simulink model "pp_sim"  (R2025a)
settings: Solver=VariableStepAuto  StartTime=0.0  StopTime=40  RelTol=1e-3
model workspace (MAT data in the model file):
  p_m = 0
  v_f = 0.8705
libraries: spsGroundLib x3, spsThreePhaseVIMeasurementLib x3, spsThreePhaseBreakerLib x3, spsSynchronousMachinepuFundamentalLib x2, spsThreePhaseProgrammableVoltageSourceLib x2, spsThreePhaseParallelRLCBranchLib x1, spsThreePhaseSourceLib x1, sps_lib x1
settings Model: Creator=reyes  LastModifiedBy=garyr

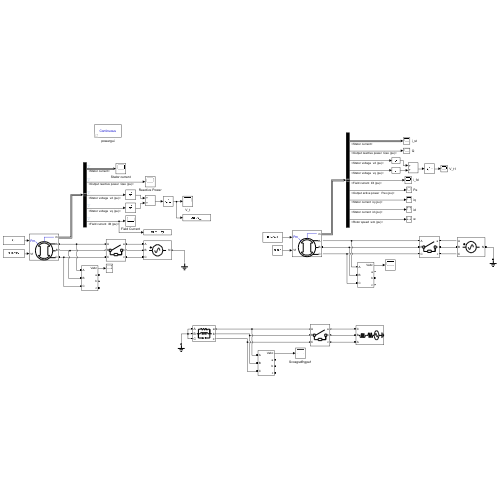
[thumbnail: Simulink's stored preview of the top-level diagram]
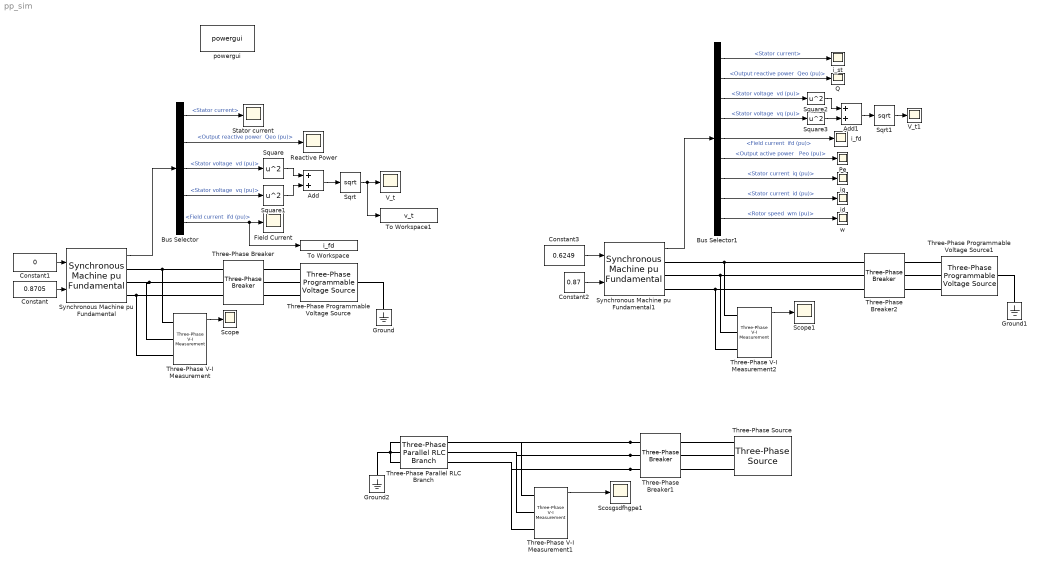
== system pp_sim ==
  Add : Sum
  Add1 : Sum
  Bus Selector : BusSelector  OutputSignals="Stator current,Output reactive power  Qeo (pu),dq0 components.Stator voltage  vd (pu),dq0 components.Stator voltage  vq (pu),dq0 components.Field current  ifd (pu)"
  Bus Selector1 : BusSelector  OutputSignals="Stator current,Output reactive power  Qeo (pu),dq0 components.Stator voltage  vd (pu),dq0 components.Stator voltage  vq (pu),dq0 components.Field current  ifd (pu),Output active power   Peo (pu),dq0 components.Stator current  iq (pu),dq0 components.Stator current  id (pu),Mechanical.Rotor speed  wm (pu)"
  Constant : Constant  Value=0.8705
  Constant1 : Constant  Tag=p_m  Value=0
  Constant2 : Constant  Value=0.87
  Constant3 : Constant  Tag=p_m  Value=0.6249
  Field Current : Scope
      settings: ActiveDisplayYMinimum=0.95426093350087715  ActiveDisplayYMaximum=0.95670423972594421  DataLoggingVariableName=ScopeData4
  Ground : spsGroundLib/Ground  LConnTagsString=a
  Ground1 : spsGroundLib/Ground  LConnTagsString=a
  Ground2 : spsGroundLib/Ground  LConnTagsString=a
  Pe : Scope
      settings: ActiveDisplayYMinimum=-266.63073278249573  ActiveDisplayYMaximum=2375.0722359085885  DataLoggingVariableName=ScopeData11
  Q : Scope
      settings: ActiveDisplayYMinimum=-0.29769400843785104  ActiveDisplayYMaximum=-0.29699694200105431  DataLoggingVariableName=ScopeData7
  Reactive Power : Scope
      settings: ActiveDisplayYMinimum=-0.1233902909232272  ActiveDisplayYMaximum=-0.12338999766576593  DataLoggingVariableName=ScopeData3
  Scope : Scope
      settings: ActiveDisplayYMinimum=-1.2502044389104019  ActiveDisplayYMaximum=1.2500642972287648  DataLoggingVariableName=ScopeData5
  Scope1 : Scope
      settings: ActiveDisplayYMinimum=-1.0713781429903637  ActiveDisplayYMaximum=0.99048701496862079  DataLoggingVariableName=ScopeData8
  Scosgsdfhgpe1 : Scope
      settings: ActiveDisplayYMinimum=-1.0092853712369843  ActiveDisplayYMaximum=1.1869510329971333  DataLoggingVariableName=ScopeData2
  Sqrt : Sqrt
  Sqrt1 : Sqrt
  Square{,1..3} (4 alike) : Math  Operator=square
  Stator current : Scope
      settings: ActiveDisplayYMinimum=0.12291954925426332  ActiveDisplayYMaximum=0.12350538497944295
  Synchronous Machine pu Fundamental : spsSynchronousMachinepuFundamentalLib/Synchronous Machine pu Fundamental  PresetModel=No  MechanicalLoad=Mechanical power Pm  ShowDetailedParameters=on  RotorType=Salient-pole  Units=per unit fundamental parameters  MeasurementBus=off  NominalParameters="[ 6250E3  4160   60]"  Stator="[ 0.00636  0.1235  0.926  0.5078 ]"  Field="[ 0.00084  0.2691]"  Dampers2=[0.0652, 0.5134, 0.0287, 0.2553, 7.765e-3, 0.9167 ]  Dampers1="[ 0.03578  0.1119  0.05366  0.1678 ]"  Mechanical=[ 7.11 0 10]  PolePairs=20  InitialConditions="[ 0  0  0  0  0  0  0  0  1 ]"  SetSaturation=off  Saturation=[0.6404,0.7127,0.8441,0.9214,0.9956,1.082,1.19,1.316,1.457;0.7,0.7698,0.8872,0.9466,0.9969,1.046,1.1,1.151,1.201]  LoadFlowParameters=[1,0,0,0,0]  TsPowergui=0  TsBlock=-1  IterativeModel=Trapezoidal non iterative  IterativeDiscreteModel=Trapezoidal non iterative  BusType=PV  Pref=0  Qref=0.3054  Qmin=-inf  Qmax=inf  PLF=0  QLF=0
      settings: LibrarySourceBlock=|
      | sps_lib/Electrical Machines/Synchronous Machine
      | pu Fundamental
  Synchronous Machine pu Fundamental1 : spsSynchronousMachinepuFundamentalLib/Synchronous Machine pu Fundamental  PresetModel=No  MechanicalLoad=Mechanical power Pm  ShowDetailedParameters=on  RotorType=Salient-pole  Units=per unit fundamental parameters  MeasurementBus=off  NominalParameters="[ 6250E3  4160   60]"  Stator="[ 0.00636  0.1235  0.926  0.5078 ]"  Field="[ 0.0084  0.2691]"  Dampers2=[0.0652, 0.5134, 0.0287, 0.2553, 7.765e-3, 0.9167 ]  Dampers1="[ 0.03578  0.1119  0.05366  0.1678 ]"  Mechanical=[ 7.11 0 20]  PolePairs=20  InitialConditions="[ 0  0  0  0  0  0  0  0  1 ]"  SetSaturation=on  Saturation=[0.6404,0.7127,0.8441,0.9214,0.9956,1.082,1.19,1.316,1.457;0.7,0.7698,0.8872,0.9466,0.9969,1.046,1.1,1.151,1.201]  LoadFlowParameters=[1,0,0,0,0]  TsPowergui=0  TsBlock=-1  IterativeModel=Trapezoidal non iterative  IterativeDiscreteModel=Trapezoidal non iterative  BusType=PQ  Pref=0.6249  Qref=0.3054  Qmin=-inf  Qmax=inf  PLF=0  QLF=0
      settings: LibrarySourceBlock=|
      | sps_lib/Electrical Machines/Synchronous Machine
      | pu Fundamental
  Three-Phase Parallel RLC Branch : spsThreePhaseParallelRLCBranchLib/Three-Phase Parallel RLC Branch  LConnTagsString=A|B|C  RConnTagsString=A|B|C  BranchType=RLC  Resistance=10  Inductance=1e-3  Capacitance=0  Measurements=None
  Three-Phase Programmable Voltage Source : spsThreePhaseProgrammableVoltageSourceLib/Three-Phase Programmable Voltage Source  PositiveSequence="[4160  0 60]"  VariationEntity=None  VariationType=Table of time-amplitude pairs  VariationTypeAlt=Step  VariationStep=0.5  VariationRate=10  VariationMagnitude=0.3  VariationFrequency=2  VariationTiming=[1 2]  VariationPhaseA=off  Amplitudes=[1 0.8 1.2 1.0]  TimeValues=[0 0.1 0.15 0.2]  HarmonicGeneration=off  HarmonicA=[3 0.2 -25 0]  HarmonicB=[2 0.15 35 2]  Timing="[0.05  3]"  BusType=PV  Pref=0  Qref=0  Qmin=-inf  Qmax=inf
  Three-Phase Programmable Voltage Source1 : spsThreePhaseProgrammableVoltageSourceLib/Three-Phase Programmable Voltage Source  PositiveSequence="[4160  0 60]"  VariationEntity=None  VariationType=Table of time-amplitude pairs  VariationTypeAlt=Step  VariationStep=0.5  VariationRate=10  VariationMagnitude=0.3  VariationFrequency=2  VariationTiming=[1 2]  VariationPhaseA=off  Amplitudes=[1 0.8 1.2 1.0]  TimeValues=[0 0.1 0.15 0.2]  HarmonicGeneration=off  HarmonicA=[3 0.2 -25 0]  HarmonicB=[2 0.15 35 2]  Timing="[0.05  3]"  BusType=PV  Pref=0  Qref=-0.3054  Qmin=-inf  Qmax=inf
  Three-Phase V-I Measurement : spsThreePhaseVIMeasurementLib/Three-Phase V-I Measurement  VoltageMeasurement=phase-to-ground  SetLabelV=off  LabelV=Vabc  Vpu=on  VpuLL=off  CurrentMeasurement=no  SetLabelI=off  LabelI=Iabc  Ipu=off  Pbase=100e6  Vbase=4160  OutputType=Complex  PhasorSimulation=off  PSBequivalent=0
  Three-Phase V-I Measurement1 : spsThreePhaseVIMeasurementLib/Three-Phase V-I Measurement  VoltageMeasurement=phase-to-ground  SetLabelV=off  LabelV=Vabc  Vpu=on  VpuLL=off  CurrentMeasurement=no  SetLabelI=off  LabelI=Iabc  Ipu=off  Pbase=100e6  Vbase=4160  OutputType=Complex  PhasorSimulation=off  PSBequivalent=0
  Three-Phase V-I Measurement2 : spsThreePhaseVIMeasurementLib/Three-Phase V-I Measurement  VoltageMeasurement=phase-to-ground  SetLabelV=off  LabelV=Vabc  Vpu=on  VpuLL=off  CurrentMeasurement=no  SetLabelI=off  LabelI=Iabc  Ipu=off  Pbase=100e6  Vbase=4160  OutputType=Complex  PhasorSimulation=off  PSBequivalent=0
  Three-Phase Breaker : spsThreePhaseBreakerLib/Three-Phase Breaker  InitialState=open  SwitchA=on  SwitchB=on  SwitchC=on  SwitchTimes="[0  25]"  External=off  BreakerResistance=0.0001  SnubberResistance=1e6  SnubberCapacitance=inf  Measurements=None
  Three-Phase Breaker1 : spsThreePhaseBreakerLib/Three-Phase Breaker  InitialState=open  SwitchA=on  SwitchB=on  SwitchC=on  SwitchTimes="[0  15]"  External=off  BreakerResistance=0.0001  SnubberResistance=1e6  SnubberCapacitance=inf  Measurements=None
  Three-Phase Breaker2 : spsThreePhaseBreakerLib/Three-Phase Breaker  InitialState=open  SwitchA=on  SwitchB=on  SwitchC=on  SwitchTimes="[0  25]"  External=off  BreakerResistance=0.0001  SnubberResistance=1e6  SnubberCapacitance=inf  Measurements=None
  Three-Phase Source : spsThreePhaseSourceLib/Three-Phase Source  InternalConnection=Yg  VoltagePhases=off  Voltage=25e3  PhaseAngle=0  Voltage_phases=[25e3 25e3 25e3]/sqrt(3)  PhaseAngles_phases=[0 -120 +120]  Frequency=60  NonIdealSource=on  SpecifyImpedance=off  Resistance=0.8929  Inductance=16.58e-3  ShortCircuitLevel=100e6  BaseVoltage=25e3  XRratio=7  BusType=swing  Pref=10e3  Qref=0  Prefabc=[10e3, 10e3, 10e3]  Qrefabc=[0, 0, 0]  Qmin=-inf  Qmax=inf
  To Workspace : ToWorkspace  VariableName=i_fd  SaveFormat=Timeseries  SampleTime=-1
  To Workspace1 : ToWorkspace  VariableName=v_t  SaveFormat=Timeseries  SampleTime=-1
  V_t : Scope
      settings: ActiveDisplayYMinimum=0.96319114292580066  ActiveDisplayYMaximum=0.99738883556627056
  V_t1 : Scope
      settings: ActiveDisplayYMinimum=0.88921384118720115  ActiveDisplayYMaximum=1.040877340760493  DataLoggingVariableName=ScopeData10
  i_fd : Scope
      settings: ActiveDisplayYMinimum=0.486166253546517  ActiveDisplayYMaximum=1.1986921425905557  DataLoggingVariableName=ScopeData6
  i_st : Scope
      settings: ActiveDisplayYMinimum=0.11664480033906652  ActiveDisplayYMaximum=0.12575316014958465  DataLoggingVariableName=ScopeData9
  id : Scope
      settings: ActiveDisplayYMinimum=-4.1747274480528285  ActiveDisplayYMaximum=9.7889132148593134  DataLoggingVariableName=ScopeData13
  iq : Scope
      settings: ActiveDisplayYMinimum=0.67354040506891022  ActiveDisplayYMaximum=0.70788681885628535  DataLoggingVariableName=ScopeData12
  powergui : sps_lib/powergui  Priority=1  SimulationMode=Continuous  SampleTime=1e-5  frequency=60  Iterations=50  frequencyindice=60  Pbase=100e6  ErrMax=1e-4  UnitsV=kV  UnitsW=MW  buscounter=0  FunctionMessages=off  echomessages=off  EnableUseOfTLC=off  CurrentSourceSwitches=off  DisableSnubberDevices=off  DisableRonSwitches=off  DisableVfSwitches=off  DisplayEquations=off  AutomaticDiscreteSolvers=off  SolverType=Tustin/Backward Euler (TBE)  Interpol=off  ExternalGateDelay=off  methode=off  Ts=100  x0status=blocks  SPID=on  SwTol=0  HookPort=off  NonlinearTolerance=1e-4  nMaxIteration=100  ContinueOnMaxIteration=off  RestoreLinks=warning  ResistiveCurrentMeasurement=off  Frange=[0:2:500]  Ylog=off  Xlog=on  ShowGrid=off  save=off  variable=ZData  structure=0  ZoomFFT=off  StartTime=0.0  cycles=1  DisplayStyle=1  fundamental=60  FreqAxis=off  MaxFrequency=1000  frequencyindicesteady=1  RmsSteady=1  display=off
  w : Scope
      settings: ActiveDisplayYMinimum=0.99793701290337811  ActiveDisplayYMaximum=1.0012660502865345  DataLoggingVariableName=ScopeData16
  wires:
  Synchronous Machine pu Fundamental/1 -> Bus Selector/1
  Bus Selector/1 -> Stator current/1  "<Stator current>"
  Bus Selector/2 -> Reactive Power/1  "<Output reactive power  Qeo (pu)>"
  Bus Selector/5 -> To Workspace/1, Field Current/1  "<Field current  ifd (pu)>"
  Three-Phase V-I Measurement/1 -> Scope/1
  Constant/1 -> Synchronous Machine pu Fundamental/2
  Constant1/1 -> Synchronous Machine pu Fundamental/1
  Bus Selector/3 -> Square/1  "<Stator voltage  vd (pu)>"
  Bus Selector/4 -> Square1/1  "<Stator voltage  vq (pu)>"
  Square/1 -> Add/1
  Square1/1 -> Add/2
  Add/1 -> Sqrt/1
  Sqrt/1 -> To Workspace1/1, V_t/1
  Three-Phase V-I Measurement1/1 -> Scosgsdfhgpe1/1
  Square2/1 -> Add1/1
  Add1/1 -> Sqrt1/1
  Sqrt1/1 -> V_t1/1
  Constant3/1 -> Synchronous Machine pu Fundamental1/1
  Bus Selector1/1 -> i_st/1  "<Stator current>"
  Square3/1 -> Add1/2
  Bus Selector1/5 -> i_fd/1  "<Field current  ifd (pu)>"
  Bus Selector1/2 -> Q/1  "<Output reactive power  Qeo (pu)>"
  Synchronous Machine pu Fundamental1/1 -> Bus Selector1/1
  Bus Selector1/3 -> Square2/1  "<Stator voltage  vd (pu)>"
  Bus Selector1/4 -> Square3/1  "<Stator voltage  vq (pu)>"
  Constant2/1 -> Synchronous Machine pu Fundamental1/2
  Three-Phase V-I Measurement2/1 -> Scope1/1
  Bus Selector1/6 -> Pe/1  "<Output active power   Peo (pu)>"
  Bus Selector1/7 -> iq/1  "<Stator current  iq (pu)>"
  Bus Selector1/8 -> id/1  "<Stator current  id (pu)>"
  Bus Selector1/9 -> w/1  "<Rotor speed  wm (pu)>"
  connections:
  Three-Phase Programmable Voltage Source/LConn1 -- Ground/LConn1
  Three-Phase Programmable Voltage Source/RConn1 -- Three-Phase Breaker/RConn1
  Three-Phase Programmable Voltage Source/RConn2 -- Three-Phase Breaker/RConn2
  Three-Phase Programmable Voltage Source/RConn3 -- Three-Phase Breaker/RConn3
  Synchronous Machine pu Fundamental/RConn1 -- Three-Phase Breaker/LConn1 -- Three-Phase V-I Measurement/LConn1
  Synchronous Machine pu Fundamental/RConn2 -- Three-Phase Breaker/LConn2 -- Three-Phase V-I Measurement/LConn2
  Synchronous Machine pu Fundamental/RConn3 -- Three-Phase V-I Measurement/LConn3 -- Three-Phase Breaker/LConn3
  Three-Phase Breaker1/LConn3 -- Three-Phase Parallel RLC Branch/RConn3 -- Three-Phase V-I Measurement1/LConn3
  Three-Phase Breaker1/LConn2 -- Three-Phase Parallel RLC Branch/RConn2 -- Three-Phase V-I Measurement1/LConn2
  Three-Phase Breaker1/LConn1 -- Three-Phase Parallel RLC Branch/RConn1 -- Three-Phase V-I Measurement1/LConn1
  Three-Phase Source/RConn3 -- Three-Phase Breaker1/RConn1
  Three-Phase Source/RConn2 -- Three-Phase Breaker1/RConn2
  Three-Phase Source/RConn1 -- Three-Phase Breaker1/RConn3
  Three-Phase Parallel RLC Branch/LConn1 -- Ground2/LConn1 -- Three-Phase Parallel RLC Branch/LConn2 -- Three-Phase Parallel RLC Branch/LConn3
  Synchronous Machine pu Fundamental1/RConn3 -- Three-Phase V-I Measurement2/LConn3 -- Three-Phase Breaker2/LConn3
  Synchronous Machine pu Fundamental1/RConn1 -- Three-Phase V-I Measurement2/LConn1 -- Three-Phase Breaker2/LConn1
  Synchronous Machine pu Fundamental1/RConn2 -- Three-Phase V-I Measurement2/LConn2 -- Three-Phase Breaker2/LConn2
  Three-Phase Programmable Voltage Source1/RConn2 -- Three-Phase Breaker2/RConn2
  Three-Phase Programmable Voltage Source1/LConn1 -- Ground1/LConn1
  Three-Phase Programmable Voltage Source1/RConn3 -- Three-Phase Breaker2/RConn3
  Three-Phase Programmable Voltage Source1/RConn1 -- Three-Phase Breaker2/RConn1
